simulink library "pathFollowingController_cl"  (R2018b)
settings: Solver=VariableStepAuto  StartTime=0.0  StopTime=10.0  RelTol=1e-3
undefined symbols (not defined in the file or in its folder): aBooth, bBooth, controlAlMat, controlSigMax, initPos, kdRollMom, kdVelAng, kpRollMom, kpVelAng, latCurve, maxBank, tauRollMom, tauVelAng
libraries: courseFollow_cl x1, setpointToOutput_cl x1
settings Model: Creator=jldanie5  LastModifiedBy=jldanie5

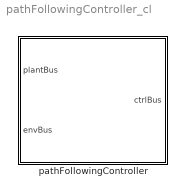
== system pathFollowingController_cl ==
  pathFollowingController : Subsystem  mask{initPosForInitSStar=initPos, searchSizeMask=pi/2, curveLatMask=latCurve, aMask=aBooth, bMask=bBooth, perpErrorValMask=3*pi/180, controlSigMaxMask=controlSigMax, maxBankMask=maxBank, controlAlMatMask=controlAlMat, kpVelAngMask=kpVelAng, kdVelAngMask=kdVelAng, tauVelAngMask=tauVelAng, kpLMask=kpRollMom, kdLMask=kdRollMom, tauLMask=tauRollMom}
      mask prompts: initPosForInitSStar "Initial Position"; searchSizeMask "Golden Section Search Size"; curveLatMask "Path Param Curve Latitude"; aMask "Path Param A"; bMask "Path Param B"; perpErrorValMask "velAng Error for 100% Perpendicular Path"; controlSigMaxMask "Maximum Control Signal"; maxBankMask "Maximum Bank Angle"; controlAlMatMask "Control Allocation Matrix"; kpVelAngMask "Vel Ang kp"; kdVelAngMask "Vel Ang kd"; tauVelAngMask "Vel Ang tau"; kpLMask "Roll Mom kp"; kdLMask "Roll Mom kd"; tauLMask "Roll Mom tau"
      mask init:
      | pathFollowingController_init
      mask DialogControl Container3 Prompt: courseFollow Params
      mask DialogControl Container4 Prompt: setpointToOutputParams

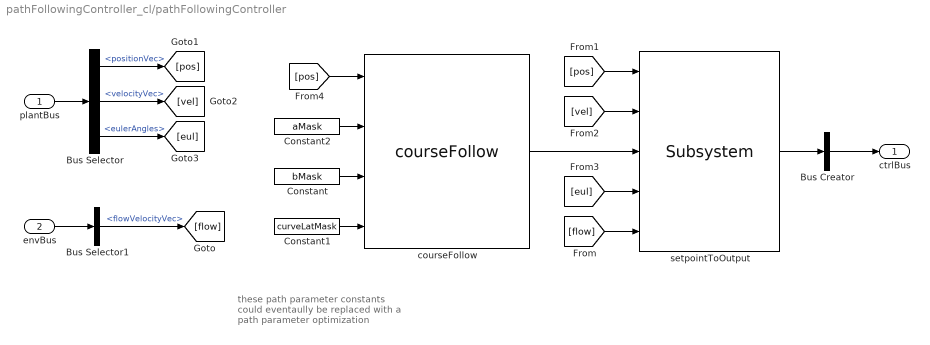
== system pathFollowingController_cl/pathFollowingController ==
  note: these path parameter constants
      | could eventaully be replaced with
      | a path parameter optimization
  plantBus : Inport  OutDataTypeStr=Bus: plantBus
  envBus : Inport  Port=2  OutDataTypeStr=Bus: envBus
  Bus Creator : BusCreator  Inputs=1  OutDataTypeStr=Bus: ctrlBus
      settings: InheritFromInputs=off
  Bus Selector : BusSelector  OutputSignals=positionVec,velocityVec,eulerAngles
  Bus Selector1 : BusSelector  OutputSignals=flowVelocityVec
  Constant : Constant  Value=bMask
  Constant1 : Constant  Value=curveLatMask
  Constant2 : Constant  Value=aMask
  courseFollow : courseFollow_cl/courseFollow  SystemSampleTime=-1
  setpointToOutput : setpointToOutput_cl/Subsystem  SystemSampleTime=-1
  ctrlBus : Outport  OutDataTypeStr=Bus: ctrlBus
  wires:
  courseFollow/1 -> setpointToOutput/3
  plantBus/1 -> Bus Selector/1
  Bus Selector/2 -> [vel]  "<velocityVec>"
  Bus Selector/1 -> [pos]  "<positionVec>"
  Bus Selector/3 -> [eul]  "<eulerAngles>"
  [pos] -> setpointToOutput/1
  [vel] -> setpointToOutput/2
  [eul] -> setpointToOutput/4
  [pos] -> courseFollow/1
  Constant2/1 -> courseFollow/2
  Constant/1 -> courseFollow/3
  Constant1/1 -> courseFollow/4
  setpointToOutput/1 -> Bus Creator/1
  Bus Creator/1 -> ctrlBus/1
  envBus/1 -> Bus Selector1/1
  Bus Selector1/1 -> [flow]  "<flowVelocityVec>"
  [flow] -> setpointToOutput/5
